simulink library "MSP_BDOT_lib"  (R2016b)
settings: Solver=VariableStepAuto  StartTime=0.0  StopTime=10.0  RelTol=1e-3
libraries: bdot_controller_lib x1
settings Model: Creator=taylorreynolds  LastModifiedBy=taylorreynolds

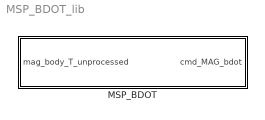
== system MSP_BDOT_lib ==
  MSP_BDOT : Subsystem

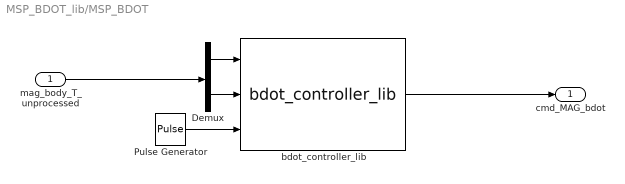
== system MSP_BDOT_lib/MSP_BDOT ==
  mag_body_T_unprocessed : Inport
  Demux : Demux  Outputs=[3 1]
  Pulse Generator : DiscretePulseGenerator  PulseType=Time based  Period=1  PulseWidth=fsw_params.actuators.magnetorquer.actuation_time_pct
  bdot_controller_lib : bdot_controller_lib/bdot_controller_lib
  cmd_MAG_bdot : Outport
  wires:
  Demux/1 -> bdot_controller_lib/1
  Demux/2 -> bdot_controller_lib/2
  mag_body_T_unprocessed/1 -> Demux/1
  bdot_controller_lib/1 -> cmd_MAG_bdot/1
  Pulse Generator/1 -> bdot_controller_lib/3
